simulink model "adcs_model"  (R2026a)
settings: Solver=VariableStepAuto
InitFcn:
  | init;
settings Model: Creator=arroy  LastModifiedBy=Owner

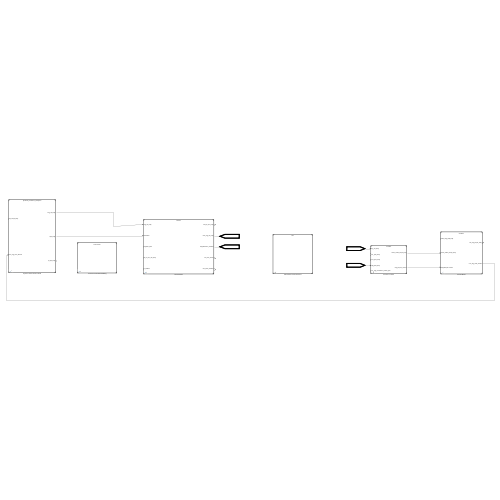
[thumbnail: Simulink's stored preview of the top-level diagram]
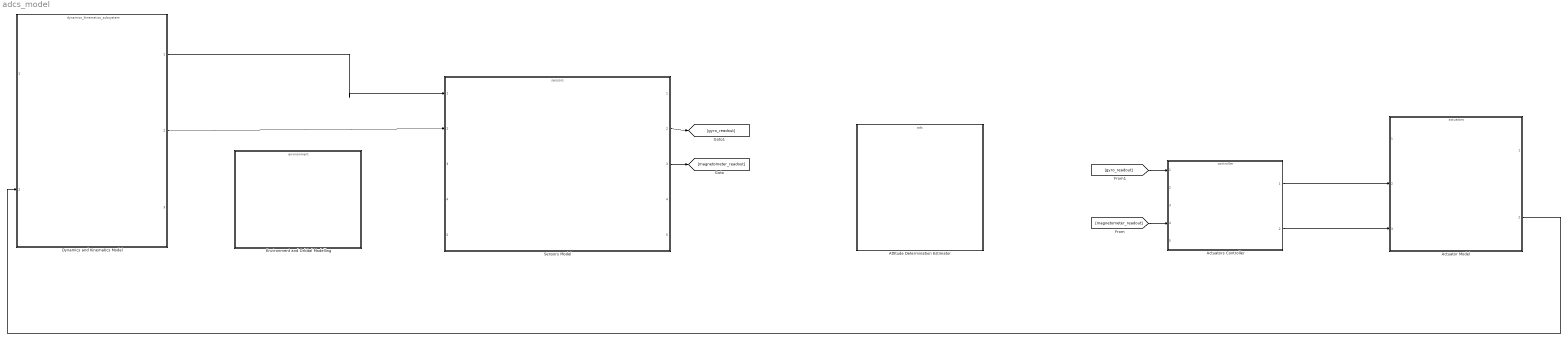
== system adcs_model ==
  Actuator Model : ModelReference  ModelNameDialog=actuators.slx  SimulationMode=Normal  ModelReferenceVersion=3.0
  Actuators Controller : ModelReference  ModelNameDialog=controller.slx  SimulationMode=Normal  ModelReferenceVersion=3.0
  Attitude Determination Estimator : ModelReference  ModelNameDialog=ads.slx  SimulationMode=Normal  ModelReferenceVersion=3.0
  Dynamics and Kinematics Model : ModelReference  ModelNameDialog=dynamics_kinematics_subsystem.slx  SimulationMode=Normal  ModelReferenceVersion=3.0
  Environment and Orbital Modelling : ModelReference  ModelNameDialog=environment.slx  SimulationMode=Normal  ModelReferenceVersion=3.0
  Sensors Model : ModelReference  ModelNameDialog=sensors.slx  SimulationMode=Normal  ModelReferenceVersion=3.0
  wires:
  Actuator Model/2 -> Dynamics and Kinematics Model/2
  Actuators Controller/1 -> Actuator Model/2
  Actuators Controller/2 -> Actuator Model/3
  Dynamics and Kinematics Model/1 -> Sensors Model/1
  Dynamics and Kinematics Model/2 -> Sensors Model/2
  Sensors Model/3 -> [magnetometer_readout]
  [magnetometer_readout] -> Actuators Controller/4
  Sensors Model/2 -> [gyro_readout]
  [gyro_readout] -> Actuators Controller/1
